simulink model "xmc_color_detection"  (R2024a)
settings: Solver=VariableStepAuto  StartTime=0.0  StopTime=inf  RelTol=1e-3
PostLoadFcn:
  | xmcHubUpdateInstalledDevice(gcs);
undefined symbols (not defined in the file or in its folder): gray, S, xc7vx485tffg1157
libraries: hlsBasic x11, color_detection_lib x8, vmcUtilities x2, dspvision x1
settings Model: Creator=ravalib  LastModifiedBy=robg
settings SolverCC: AlgebraicLoopSolver=TrustRegion
settings DataIOCC: ReturnWorkspaceOutputs=off
settings OptimizationCC: LifeSpan=inf
settings DebuggingCC: InheritedTsInSrcMsg=none  UnconnectedInputMsg=warning  UnconnectedOutputMsg=warning  UnconnectedLineMsg=warning  ArithmeticOperatorsInVariantConditions=warning
settings ModelReferenceCC: EnableRefExpFcnMdlSchedulingChecks=on
settings SFSimCC: SimUseLocalCustomCode=off  CustomCodeUndefinedFunction=UseInterfaceOnly
settings RTWCC: RTWUseLocalCustomCode=off  GPUComputeCapability=3.5  DLArmComputeVersion=19.05
settings CodeAppCC: StateflowObjectComments=on
settings ConfigComp: CovBoundaryAbsTol=1.0e-5

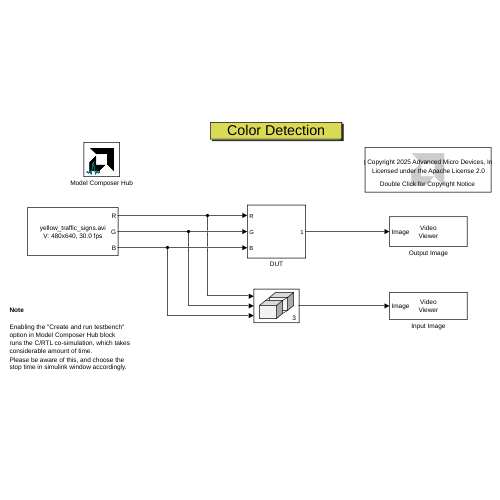
[thumbnail: Simulink's stored preview of the top-level diagram]
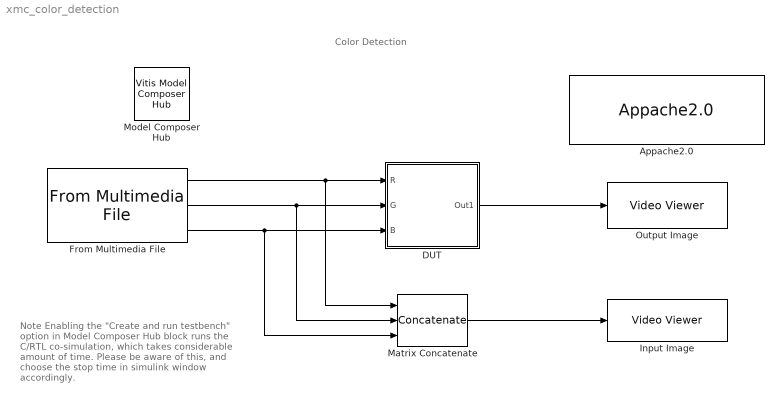
== system xmc_color_detection ==
  note: Color Detection
  note: Note
      |
      | Enabling the "Create and run testbench" option in Model Composer Hub block
      | runs the C/RTL co-simulation, which takes considerable amount of time.
      | Please be aware of this, and choose the stop time in simulink window accordingly.
  Appache2.0 : vmcUtilities/Appache2.0
  DUT : Subsystem
  From Multimedia File : dspvision/From Multimedia File  inputFilename=yellow_traffic_signs.avi  readRange=[1 Inf]  loop=on  numPlays=inf  outputStreams=Video only  videoDataType=uint8  audioDataType=int16  inheritSampleTime=off  userDefinedSampleTime=1/30  noAudioOutput=off  isIntensityVideo=off  fourcc=RGB  colorVideoFormat=Separate color signals  outputEOF=off  dataOrg=Column-major  audioFrameSize=1024  computeAudioFrameSize=off  outSamplingMode=Sample based
  Input Image : VideoViewer  colormapValue=gray(256)  FigPos=[425 718 1006 554]
  Matrix Concatenate : Concatenate  NumInputs=3  Mode=Multidimensional array  ConcatenateDimension=3
  Model Composer Hub : vmcUtilities/Vitis Model Composer Hub  Tag=genX  CodeGeneration=off  SubsystemName=DUT  BlockHierPath=xmc_color_detection/DUT  SubsystemType=HLSNode  StartColumn=1  NumberOfColumns=1  TargetDirectory=./code  exportDesign=on  analyzeDesign=off  validateDesignOnHw=off  ExportType=IP Catalog  IpVendor=xilinx.com  IpLibrary=hls  IpVersion=1.0  IpHWLanguage=Verilog  AieCompilerOptions={}  AieSimulatorOptions={}  CreateTestbench=off  TestbenchStackSize=10  RunRtlSim=off  RunCSim=off  RunAieSim=off  AieSimTimeout=50000  RunAieSimProfiling=off  LaunchVitisAnalyzer=off  PlotOutput=off  RunX86Sim=on  X86SimTimeout=10  GenHwImage=off  GenLibadfXo=off  GenHwValidationCode=off  PlatformType=Specify Platform  Platform=/proj/xbuilds/SWIP/9999.0_0818_1732/installs/lin64/2025.2/Vitis/base_platforms/xilinx_vck190_base_202520_1/xilinx_vck190_base_202520_1.xpfm  HwSystemType=Baremetal  HwValidationTarget=hw  ProjDevice=xc7vx485tffg1157-1  ProjDevicePart=xc7vx485tffg1157-1  AIEType=AIE  SamplePeriod=-1  ClockFrequency=200  DataPathParallelism=1  xilinxfamily=versalaicore  part=xcvc1902  speed=-2MP-e-S  package=vsva2197  directory=./netlist  testbench=off  incr_netlist=off  synthesis_tool=Vivado  clock_wrapper=Clock Enables  dbl_ovrd=According to Block Masks  dcm_input_clock_period=10  sysclk_period=10  simulink_period=1  eval_field=0  IPInfoJsonString="{\"DUTSubsystemName\":\"DUT\",\"HLSSubsystem\":{\"SubsystemName\":\"DUT\",\"FpgaClockFreq\":\"200\",\"IPName\":\"DUT\",\"IPLibrary\":\"hls\",\"TargetDirectory\":\"./code\"},\"SubsystemTag\":\"HLSNode\"}"  LogFileName=/proj/xhdhdstaff5/sdegala/Head1/HEAD/VMC_2025_2_July/Examples/HLS/color_detection/code/model_composer.log  NThreads=4  IPConfigFile=/tmp/vmctmp-6835010160091439353/xmc_color_detection_ipconfig.json
  Output Image : VideoViewer  colormapValue=gray(256)  FigPos=[33 747 919 556]
  wires:
  Matrix Concatenate/1 -> Input Image/1
  From Multimedia File/1 -> DUT/1(R), Matrix Concatenate/1
  From Multimedia File/2 -> DUT/2(G), Matrix Concatenate/2
  From Multimedia File/3 -> DUT/3(B), Matrix Concatenate/3
  DUT/1(Out1) -> Output Image/1

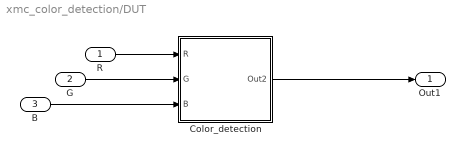
== system xmc_color_detection/DUT ==
  R : Inport
  G : Inport  Port=2
  B : Inport  Port=3
  Color_detection : Subsystem
      mask Display: xmcDrawBlockIcon();
  Out1 : Outport
  wires:
  Color_detection/1(Out2) -> Out1/1
  R/1 -> Color_detection/1(R)
  B/1 -> Color_detection/3(B)
  G/1 -> Color_detection/2(G)

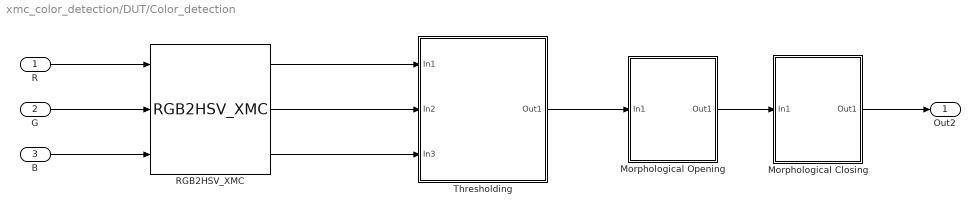
== system xmc_color_detection/DUT/Color_detection ==
  R : Inport
  G : Inport  Port=2
  B : Inport  Port=3
  Morphological Closing : Subsystem
      mask Display: xmcDrawBlockIcon();
  Morphological Opening : Subsystem
      mask Display: xmcDrawBlockIcon();
  RGB2HSV_XMC : color_detection_lib/RGB2HSV_XMC  LibraryFunction=RGB2HSV_XMC  IncludeFiles={'RGB2HSV_wrap.h'}  SourceFiles={}  IncludeDirectories={'./include'}  TemplateParams={'int ROWS'; 'int COLS'}  FunctionParamTypes={xmcDataType('void'); xmcDataType('uint8_t'); xmcDataType('uint8_t'); xmcDataType('uint8_t'); xmcDataType('uint8_t'); xmcDataType('uint8_t'); xmcDataType('uint8_t')}  FunctionParamPassbys={0.000000000000000000e+00; 0.000000000000000000e+00; 0.000000000000000000e+00; 0.000000000000000000e+00; 0.000000000000000000e+00; 0.000000000000000000e+00; 0.000000000000000000e+00}  FunctionParamDimensions={'1'; '[ROWS][COLS]'; '[ROWS][COLS]'; '[ROWS][COLS]'; '[ROWS][COLS]'; '[ROWS][COLS]'; '[ROWS][COLS]'}  FunctionParamNames={'return'; 'R'; 'G'; 'B'; 'H'; 'S'; 'V'}  FunctionParamDir={0.000000000000000000e+00; 1.000000000000000000e+00; 1.000000000000000000e+00; 1.000000000000000000e+00; 2.000000000000000000e+00; 2.000000000000000000e+00; 2.000000000000000000e+00}  FunctionParamSupportsStreaming={true; true; true; true; true; true; true}  BufferDepth={'0'}  FunctionParamValues={'0'; '0'; '0'; '0'; '0'; '0'; '0'}  ThroughputFactors={''}
  Thresholding : Subsystem  mask(Color Threshold){hue_low=20, hue_high=31, saturation_low=128, saturation_high=255, value_low=128, value_high=255}
      mask prompts: hue_low "Hue Low"; hue_high "Hue High"; saturation_low "Saturation Low"; saturation_high "Saturation High"; value_low "Value Low"; value_high "Value High"
      mask help: Compares the Hue, Saturation, and Value channels to the specificed threholds and renders a binary image.
      mask Help: Threshold Values should be between 0 and 255 inclusive. Use a phot editor tool to get the thresholds.
      mask DialogControl ParameterGroupVar Prompt: HSV Thresholds
      mask Display: xmcDrawBlockIcon();
  Out2 : Outport
  wires:
  RGB2HSV_XMC/2 -> Thresholding/2(In2)
  G/1 -> RGB2HSV_XMC/2
  Thresholding/1(Out1) -> Morphological Opening/1(In1)
  Morphological Opening/1(Out1) -> Morphological Closing/1(In1)
  Morphological Closing/1(Out1) -> Out2/1
  B/1 -> RGB2HSV_XMC/3
  R/1 -> RGB2HSV_XMC/1
  RGB2HSV_XMC/1 -> Thresholding/1(In1)
  RGB2HSV_XMC/3 -> Thresholding/3(In3)

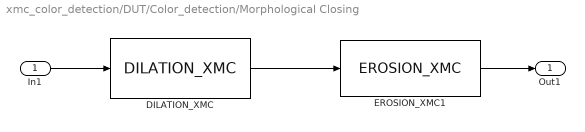
== system xmc_color_detection/DUT/Color_detection/Morphological Closing ==
  In1 : Inport
  DILATION_XMC : color_detection_lib/DILATION_XMC  LibraryFunction=DILATION_XMC  IncludeFiles={'DILATION_wrap.h'}  SourceFiles={}  IncludeDirectories={'./include'}  TemplateParams={'int ROWS'; 'int COLS'}  FunctionParamTypes={xmcDataType('void'); xmcDataType('uint8_t'); xmcDataType('uint8_t'); xmcDataType('unsigned char')}  FunctionParamPassbys={0.000000000000000000e+00; 0.000000000000000000e+00; 0.000000000000000000e+00; 0.000000000000000000e+00}  FunctionParamDimensions={'1'; '[ROWS][COLS]'; '[ROWS][COLS]'; '[9]'}  FunctionParamNames={'return'; 'src'; 'dst'; 'kernel'}  FunctionParamDir={0.000000000000000000e+00; 1.000000000000000000e+00; 2.000000000000000000e+00; 3.000000000000000000e+00}  FunctionParamSupportsStreaming={true; true; true; true}  BufferDepth={'0'}  FunctionParamValues={'0'; '0'; '0'; '0'}  ThroughputFactors={''}  kernel=[1 1 1 1 1 1 1 1 1]
  EROSION_XMC1 : color_detection_lib/EROSION_XMC  LibraryFunction=EROSION_XMC  IncludeFiles={'EROSION_wrap.h'}  SourceFiles={}  IncludeDirectories={'./include'}  TemplateParams={'int ROWS'; 'int COLS'}  FunctionParamTypes={xmcDataType('void'); xmcDataType('uint8_t'); xmcDataType('uint8_t'); xmcDataType('unsigned char')}  FunctionParamPassbys={0.000000000000000000e+00; 0.000000000000000000e+00; 0.000000000000000000e+00; 0.000000000000000000e+00}  FunctionParamDimensions={'1'; '[ROWS][COLS]'; '[ROWS][COLS]'; '[9]'}  FunctionParamNames={'return'; 'src'; 'dst'; 'kernel'}  FunctionParamDir={0.000000000000000000e+00; 1.000000000000000000e+00; 2.000000000000000000e+00; 3.000000000000000000e+00}  FunctionParamSupportsStreaming={true; true; true; true}  BufferDepth={'0'}  FunctionParamValues={'0'; '0'; '0'; '0'}  ThroughputFactors={''}  kernel=[1 1 1 1 1 1 1 1 1]
  Out1 : Outport
  wires:
  DILATION_XMC/1 -> EROSION_XMC1/1
  In1/1 -> DILATION_XMC/1
  EROSION_XMC1/1 -> Out1/1

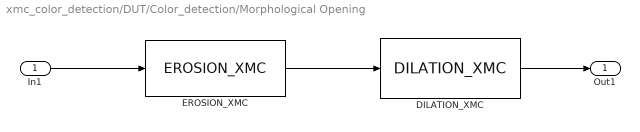
== system xmc_color_detection/DUT/Color_detection/Morphological Opening ==
  In1 : Inport
  DILATION_XMC : color_detection_lib/DILATION_XMC  LibraryFunction=DILATION_XMC  IncludeFiles={'DILATION_wrap.h'}  SourceFiles={}  IncludeDirectories={'./include'}  TemplateParams={'int ROWS'; 'int COLS'}  FunctionParamTypes={xmcDataType('void'); xmcDataType('uint8_t'); xmcDataType('uint8_t'); xmcDataType('unsigned char')}  FunctionParamPassbys={0.000000000000000000e+00; 0.000000000000000000e+00; 0.000000000000000000e+00; 0.000000000000000000e+00}  FunctionParamDimensions={'1'; '[ROWS][COLS]'; '[ROWS][COLS]'; '[9]'}  FunctionParamNames={'return'; 'src'; 'dst'; 'kernel'}  FunctionParamDir={0.000000000000000000e+00; 1.000000000000000000e+00; 2.000000000000000000e+00; 3.000000000000000000e+00}  FunctionParamSupportsStreaming={true; true; true; true}  BufferDepth={'0'}  FunctionParamValues={'0'; '0'; '0'; '0'}  ThroughputFactors={''}  kernel=[1 1 1 1 1 1 1 1 1]
  EROSION_XMC : color_detection_lib/EROSION_XMC  LibraryFunction=EROSION_XMC  IncludeFiles={'EROSION_wrap.h'}  SourceFiles={}  IncludeDirectories={'./include'}  TemplateParams={'int ROWS'; 'int COLS'}  FunctionParamTypes={xmcDataType('void'); xmcDataType('uint8_t'); xmcDataType('uint8_t'); xmcDataType('unsigned char')}  FunctionParamPassbys={0.000000000000000000e+00; 0.000000000000000000e+00; 0.000000000000000000e+00; 0.000000000000000000e+00}  FunctionParamDimensions={'1'; '[ROWS][COLS]'; '[ROWS][COLS]'; '[9]'}  FunctionParamNames={'return'; 'src'; 'dst'; 'kernel'}  FunctionParamDir={0.000000000000000000e+00; 1.000000000000000000e+00; 2.000000000000000000e+00; 3.000000000000000000e+00}  FunctionParamSupportsStreaming={true; true; true; true}  BufferDepth={'0'}  FunctionParamValues={'0'; '0'; '0'; '0'}  ThroughputFactors={''}  kernel=[1 1 1 1 1 1 1 1 1]
  Out1 : Outport
  wires:
  EROSION_XMC/1 -> DILATION_XMC/1
  In1/1 -> EROSION_XMC/1
  DILATION_XMC/1 -> Out1/1

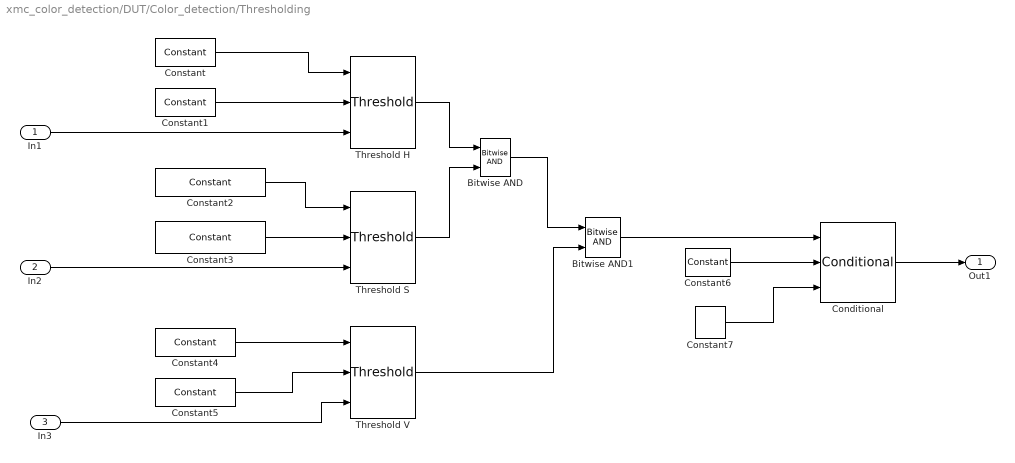
== system xmc_color_detection/DUT/Color_detection/Thresholding ==
  In1 : Inport
  In2 : Inport  Port=2
  In3 : Inport  Port=3
  Bitwise AND : hlsBasic/Bitwise AND
  Bitwise AND1 : hlsBasic/Bitwise AND
  Conditional : hlsBasic/Conditional  Condition=C ~= 0  Threshold=0.00
  Constant : hlsBasic/Constant  Value=hue_low  VectorParams1D=off  SampleTime=-1  OutDataType=uint8  TypeExp=''  Signedness=Signed  WordLength=16  FractionalLength=0  RoundingMode=Truncation to minus infinity  OverflowMode=Wrap around
  Constant1 : hlsBasic/Constant  Value=hue_high  VectorParams1D=off  SampleTime=-1  OutDataType=uint8  TypeExp=''  Signedness=Signed  WordLength=16  FractionalLength=0  RoundingMode=Truncation to minus infinity  OverflowMode=Wrap around
  Constant2 : hlsBasic/Constant  Value=saturation_low  VectorParams1D=off  SampleTime=-1  OutDataType=uint8  TypeExp=''  Signedness=Signed  WordLength=16  FractionalLength=0  RoundingMode=Truncation to minus infinity  OverflowMode=Wrap around
  Constant3 : hlsBasic/Constant  Value=saturation_high  VectorParams1D=off  SampleTime=-1  OutDataType=uint8  TypeExp=''  Signedness=Signed  WordLength=16  FractionalLength=0  RoundingMode=Truncation to minus infinity  OverflowMode=Wrap around
  Constant4 : hlsBasic/Constant  Value=value_low  VectorParams1D=off  SampleTime=-1  OutDataType=uint8  TypeExp=''  Signedness=Signed  WordLength=16  FractionalLength=0  RoundingMode=Truncation to minus infinity  OverflowMode=Wrap around
  Constant5 : hlsBasic/Constant  Value=value_high  VectorParams1D=off  SampleTime=-1  OutDataType=uint8  TypeExp=''  Signedness=Signed  WordLength=16  FractionalLength=0  RoundingMode=Truncation to minus infinity  OverflowMode=Wrap around
  Constant6 : hlsBasic/Constant  Value=1  VectorParams1D=off  SampleTime=-1  OutDataType=uint8  TypeExp=''  Signedness=Signed  WordLength=16  FractionalLength=0  RoundingMode=Truncation to minus infinity  OverflowMode=Wrap around
  Constant7 : hlsBasic/Constant  Value=0  VectorParams1D=off  SampleTime=-1  OutDataType=uint8  TypeExp=''  Signedness=Signed  WordLength=16  FractionalLength=0  RoundingMode=Truncation to minus infinity  OverflowMode=Wrap around
  Threshold H : color_detection_lib/Threshold  SystemSampleTime=-1  VariantActivationTime=update diagram  EmptyChoice=off  PassThrough=off  PassThroughVariantControl=(default)  EmptyChoiceVariantControl=(default)  AllowFlexibleInterface=on  Latency=0  AutoFrameSizeCalculation=off
  Threshold S : color_detection_lib/Threshold  SystemSampleTime=-1  VariantActivationTime=update diagram  EmptyChoice=off  PassThrough=off  PassThroughVariantControl=(default)  EmptyChoiceVariantControl=(default)  AllowFlexibleInterface=on  Latency=0  AutoFrameSizeCalculation=off
  Threshold V : color_detection_lib/Threshold  SystemSampleTime=-1  VariantActivationTime=update diagram  EmptyChoice=off  PassThrough=off  PassThroughVariantControl=(default)  EmptyChoiceVariantControl=(default)  AllowFlexibleInterface=on  Latency=0  AutoFrameSizeCalculation=off
  Out1 : Outport
  wires:
  Conditional/1 -> Out1/1
  Bitwise AND1/1 -> Conditional/1
  Constant6/1 -> Conditional/2
  Constant7/1 -> Conditional/3
  Threshold S/1 -> Bitwise AND/2
  Constant5/1 -> Threshold V/2
  In2/1 -> Threshold S/3
  Constant2/1 -> Threshold S/1
  Threshold V/1 -> Bitwise AND1/2
  In3/1 -> Threshold V/3
  Threshold H/1 -> Bitwise AND/1
  Constant3/1 -> Threshold S/2
  In1/1 -> Threshold H/3
  Constant4/1 -> Threshold V/1
  Bitwise AND/1 -> Bitwise AND1/1
  Constant1/1 -> Threshold H/2
  Constant/1 -> Threshold H/1
